simulink model "decentralized_LQR"  (R2021b)
settings: Solver=FixedStepDiscrete  StartTime=0.0  StopTime=600  FixedStep=0.5  RelTol=1e-3
values from neighbouring files (symbols this model uses):
  cte = quadrupleLoadParameters()    [decentralizedLQRComputeEqMatrices.m]
undefined symbols (not defined in the file or in its folder): cteLQR, DiscIntNeverNeededParam
libraries: sldrtlib x1
settings Model: SimulationMode=accelerator  Creator=IST  LastModifiedBy=IST

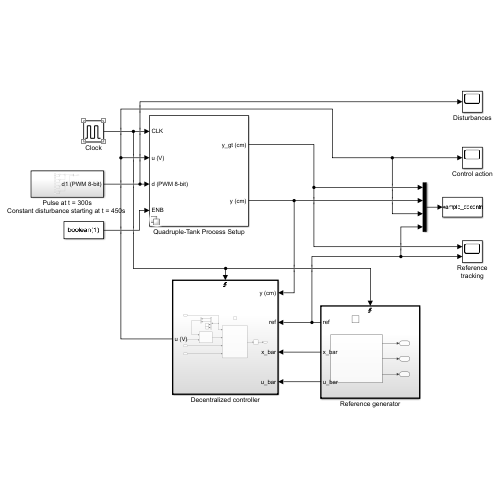
[thumbnail: Simulink's stored preview of the top-level diagram]
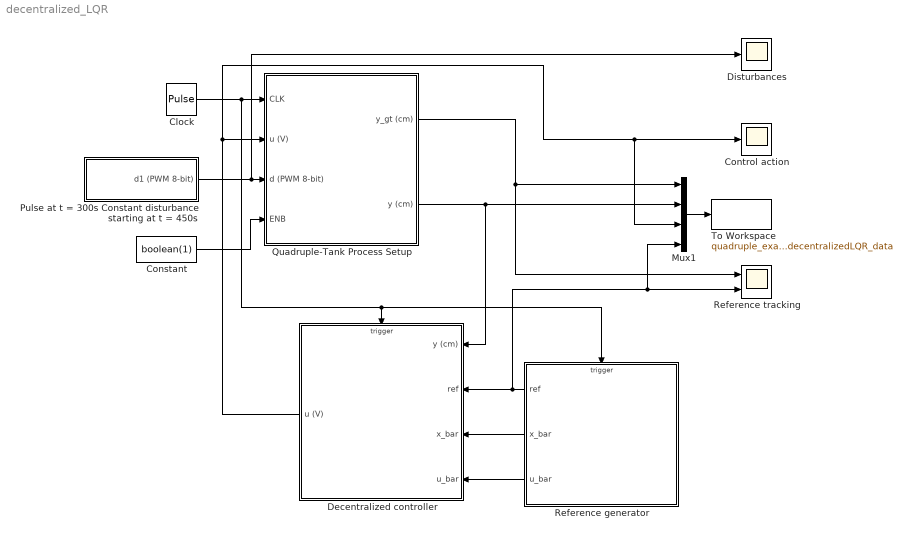
== system decentralized_LQR ==
  Clock : DiscretePulseGenerator  PulseType=Time based  Period=1  PulseWidth=50
  Constant : Constant  Priority=4  Value=boolean(1)
  Control action : Scope
      settings: Priority=20
  Decentralized controller : Subsystem  Priority=3  InitFcn=|
      | decentralizedLQRComputeEqMatrices();
      | cteLQR = decentralizedLQRLoadParameters();
  Disturbances : Scope
  Mux1 : Mux
  "Pulse at t = 300s Constant disturbance starting at t = 450s " : Subsystem
  Quadruple-Tank Process Setup : Subsystem  InitFcn=|  StopFcn=|  Variant=on
      InitFcn=|
      | % Load parameters
      | cte = quadrupleLoadParameters();
      | % Select simulation mode if unspecified
      | if ~exist('experimentalSetup')
      | experimentalSetup = false;
      | end
      | if experimentalSetup
      | if exist('arduinoPort')
      | arduino = serial(arduinoPort,...
      |                 'BaudRate',9600,...
      |                 'ByteOrder','bigEndian',...
      |                 'DataBits',8,...
      |                 'StopBits',1,...
      |                 'Terminator','');
      | arduino.Parity = 'none';
      | fopen(arduino);
      | else
      | error("Error: Arduino port undefined. Define the port in workspace variable 'arduinoPort'.");
      | end
      | end
      StopFcn=|
      | if experimentalSetup
      | fclose(arduino);
      | end
  Reference tracking : Scope  NumInputPorts=2
      settings: Priority=20
  Reference generator : Subsystem  Priority=2
  To Workspace : ToWorkspace  VariableName=quadruple_example_decentralizedLQR_data  SaveFormat=Timeseries  SampleTime=1
      settings: Priority=20
  wires:
  Quadruple-Tank Process Setup/1(y_gt (cm)) -> Reference tracking/1, Mux1/1
  Clock/1 -> Quadruple-Tank Process Setup/1(CLK), Reference generator/Trigger, Decentralized controller/Trigger
  Quadruple-Tank Process Setup/2(y (cm)) -> Decentralized controller/1(y (cm)), Mux1/2
  Mux1/1 -> To Workspace/1
  Reference generator/3(u_bar) -> Decentralized controller/4(u_bar)
  "Pulse at t = 300s Constant disturbance starting at t = 450s "/1(d1 (PWM 8-bit)) -> Disturbances/1, Quadruple-Tank Process Setup/3(d (PWM 8-bit))
  Constant/1 -> Quadruple-Tank Process Setup/4(ENB)
  Decentralized controller/1(u (V)) -> Quadruple-Tank Process Setup/2(u (V)), Mux1/3, Control action/1
  Reference generator/2(x_bar) -> Decentralized controller/3(x_bar)
  Reference generator/1(ref) -> Decentralized controller/2(ref), Mux1/4, Reference tracking/2

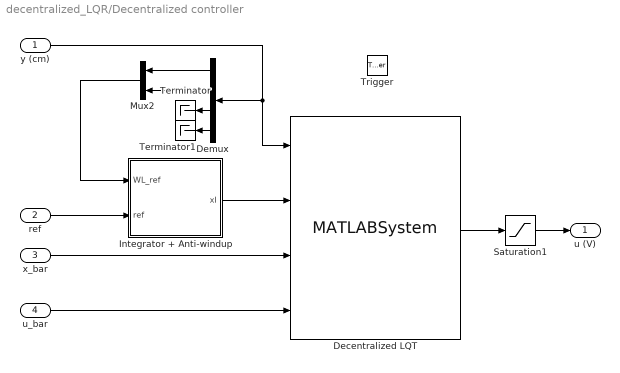
== system decentralized_LQR/Decentralized controller ==
  y (cm) : Inport
  ref : Inport  Port=2
  x_bar : Inport  Port=3
  u_bar : Inport  Port=4
  Trigger : TriggerPort  VariantControl=Variant  PortDimensions=1
  Decentralized LQT : MATLABSystem  System=controllerObj  dT=cteLQR.dT  T=cteLQR.T  d=cteLQR.d  SimulateUsing=Code generation
      mask Type: controllerObj
      mask Display:
      | disp('controllerObj');
      | port_label('input',1,'WL');
      | port_label('input',2,'xI');
      | port_label('input',3,'x_bar');
      | port_label('input',4,'u_bar');
      | port_label('output',1,'u');
  Demux : Demux
  Integrator + Anti-windup : Subsystem
  Mux2 : Mux  Inputs=2
  Saturation1 : Saturate  UpperLimit=cteLQR.uMax  LowerLimit=cteLQR.uMin
  Terminator : Terminator
  Terminator1 : Terminator
  u (V) : Outport  VectorParamsAs1DForOutWhenUnconnected=off
  wires:
  Demux/2 -> Mux2/2
  Demux/3 -> Terminator/1
  Integrator + Anti-windup/1(xI) -> Decentralized LQT/2
  Mux2/1 -> Integrator + Anti-windup/1(WL_ref)
  y (cm)/1 -> Decentralized LQT/1, Demux/1
  ref/1 -> Integrator + Anti-windup/2("ref ")
  Decentralized LQT/1 -> Saturation1/1
  Demux/1 -> Mux2/1
  Demux/4 -> Terminator1/1
  Saturation1/1 -> u (V)/1
  u_bar/1 -> Decentralized LQT/4
  x_bar/1 -> Decentralized LQT/3

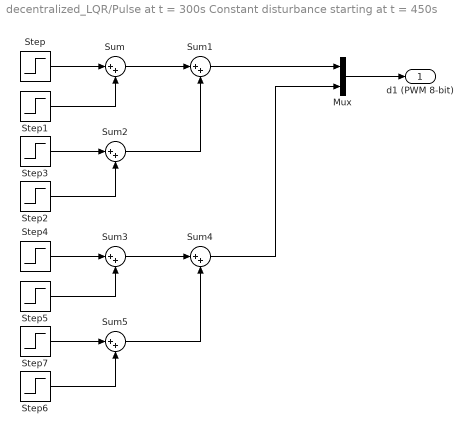
== system decentralized_LQR/Pulse at t = 300s Constant disturbance starting at t = 450s  ==
  Mux : Mux  Inputs=2
  Step : Step  Time=300  After=50  SampleTime=0
  Step1 : Step  Time=304  After=-50  SampleTime=0
  Step2 : Step  Time=451  After=-41  SampleTime=0
  Step3 : Step  Time=450  After=50  SampleTime=0
  Step4 : Step  Time=250  After=50  SampleTime=0
  Step5 : Step  Time=254  After=-50  SampleTime=0
  Step6 : Step  Time=401  After=-41  SampleTime=0
  Step7 : Step  Time=400  After=50  SampleTime=0
  Sum{,1..5} (6 alike) : Sum  Inputs=|++
  d1 (PWM 8-bit) : Outport  VectorParamsAs1DForOutWhenUnconnected=off
  wires:
  Step/1 -> Sum/1
  Step1/1 -> Sum/2
  Sum/1 -> Sum1/1
  Step3/1 -> Sum2/1
  Step2/1 -> Sum2/2
  Sum2/1 -> Sum1/2
  Sum1/1 -> Mux/1
  Step6/1 -> Sum5/2
  Step4/1 -> Sum3/1
  Sum5/1 -> Sum4/2
  Step5/1 -> Sum3/2
  Step7/1 -> Sum5/1
  Sum4/1 -> Mux/2
  Sum3/1 -> Sum4/1
  Mux/1 -> d1 (PWM 8-bit)/1

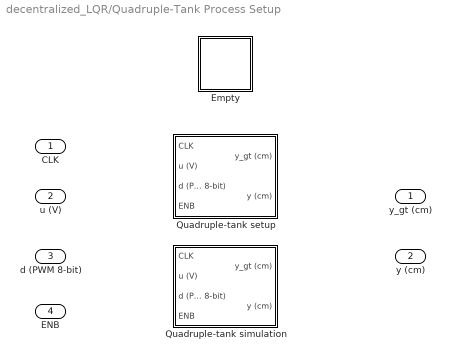
== system decentralized_LQR/Quadruple-Tank Process Setup ==
  CLK : Inport
  u (V) : Inport  Port=2
  d (PWM 8-bit) : Inport  Port=3
  ENB : Inport  Port=4
  Empty : Subsystem  VariantControl=%
  Quadruple-tank setup : Subsystem  VariantControl=experimentalSetup == true
  Quadruple-tank simulation : Subsystem  Priority=4  VariantControl=experimentalSetup == false
  y_gt (cm) : Outport  VectorParamsAs1DForOutWhenUnconnected=off
  y (cm) : Outport  Port=2  VectorParamsAs1DForOutWhenUnconnected=off

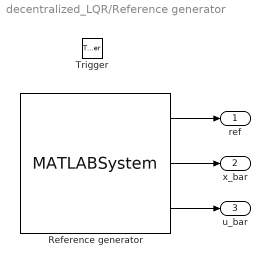
== system decentralized_LQR/Reference generator ==
  Trigger : TriggerPort  VariantControl=Variant  PortDimensions=1
  Reference generator : MATLABSystem  System=referenceGenerator  dT=cteLQR.dT  T=cteLQR.T  SimulateUsing=Code generation  Waveform1=Sin  Period1=400  Amplitude1=5  Bias1=13  Phase1=0  Waveform2=Square  Period2=300  Amplitude2=5  Bias2=13  Phase2=0
      mask Type: referenceGenerator
      mask Display:
      | disp('referenceGenerator');
      | port_label('output',1,'ref');
      | port_label('output',2,'x_bar');
      | port_label('output',3,'u_bar');
  ref : Outport  VectorParamsAs1DForOutWhenUnconnected=off
  x_bar : Outport  Port=2  VectorParamsAs1DForOutWhenUnconnected=off
  u_bar : Outport  Port=3  VectorParamsAs1DForOutWhenUnconnected=off
  wires:
  Reference generator/1 -> ref/1
  Reference generator/3 -> u_bar/1
  Reference generator/2 -> x_bar/1

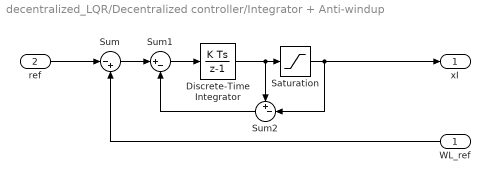
== system decentralized_LQR/Decentralized controller/Integrator + Anti-windup ==
  WL_ref : Inport
  "ref " : Inport  Port=2
  Discrete-Time Integrator : DiscreteIntegrator  SampleTime=-1  ICPrevOutput=DiscIntNeverNeededParam  ICPrevScaledInput=DiscIntNeverNeededParam
  Saturation : Saturate  UpperLimit=cteLQR.AntiWU  LowerLimit=-cteLQR.AntiWU
  Sum : Sum  Inputs=|-+
  Sum1 : Sum  Inputs=|+-
  Sum2 : Sum  Inputs=+-|
  xI : Outport  VectorParamsAs1DForOutWhenUnconnected=off
  wires:
  Discrete-Time Integrator/1 -> Sum2/1, Saturation/1
  "ref "/1 -> Sum/1
  WL_ref/1 -> Sum/2
  Sum2/1 -> Sum1/2
  Saturation/1 -> xI/1, Sum2/2
  Sum1/1 -> Discrete-Time Integrator/1
  Sum/1 -> Sum1/1

== system decentralized_LQR/Quadruple-Tank Process Setup/Empty ==

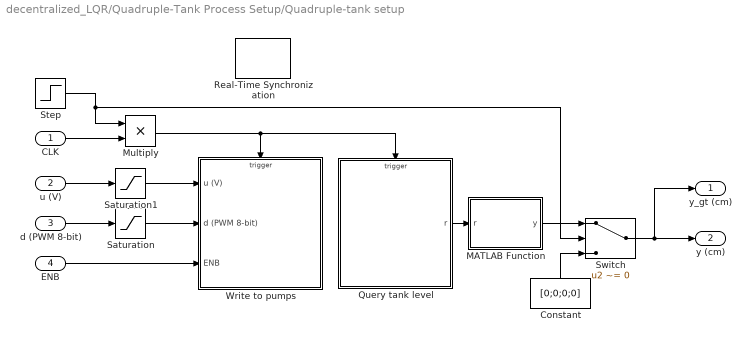
== system decentralized_LQR/Quadruple-Tank Process Setup/Quadruple-tank setup ==
  CLK : Inport
  u (V) : Inport  Port=2
  d (PWM 8-bit) : Inport  Port=3
  ENB : Inport  Port=4
  Constant : Constant  Value=[0;0;0;0]
  MATLAB Function : MATLAB Function  TreatAsAtomicUnit=on
  Multiply : Product
  Query tank level : Subsystem  Priority=1
  Real-Time Synchronization : sldrtlib/Real-Time Synchronization  Priority=5  SampleTime=0.5  MaxMissedTicks=10  ShowMissedTicks=off  YieldWhenWaiting=off
  Saturation : Saturate  UpperLimit=255  LowerLimit=0
  Saturation1 : Saturate  UpperLimit=cte.uMax  LowerLimit=cte.uMin
  Step : Step  Time=5  SampleTime=0
  Switch : Switch  Criteria=u2 ~= 0
  Write to pumps : Subsystem  Priority=100
  y_gt (cm) : Outport  VectorParamsAs1DForOutWhenUnconnected=off
  y (cm) : Outport  Port=2  VectorParamsAs1DForOutWhenUnconnected=off
  wires:
  ENB/1 -> Write to pumps/3(ENB)
  Query tank level/1(r) -> MATLAB Function/1(r)
  d (PWM 8-bit)/1 -> Saturation/1
  Saturation/1 -> Write to pumps/2(d (PWM 8-bit))
  u (V)/1 -> Saturation1/1
  Saturation1/1 -> Write to pumps/1(u (V))
  MATLAB Function/1(y) -> Switch/1
  Switch/1 -> y_gt (cm)/1, y (cm)/1
  Constant/1 -> Switch/3
  Step/1 -> Multiply/1, Switch/2
  CLK/1 -> Multiply/2
  Multiply/1 -> Write to pumps/Trigger, Query tank level/Trigger

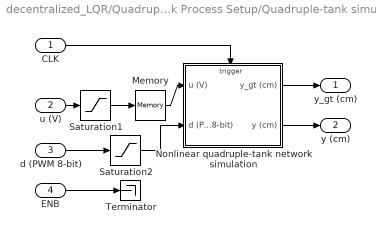
== system decentralized_LQR/Quadruple-Tank Process Setup/Quadruple-tank simulation ==
  CLK : Inport
  u (V) : Inport  Port=2
  d (PWM 8-bit) : Inport  Port=3
  ENB : Inport  Port=4
  Memory : Memory
  Nonlinear quadruple-tank network simulation : Subsystem  Priority=10
  Saturation1 : Saturate  UpperLimit=cte.uMax  LowerLimit=cte.uMin
  Saturation2 : Saturate  UpperLimit=2^8-1  LowerLimit=0
  Terminator : Terminator
  y_gt (cm) : Outport  VectorParamsAs1DForOutWhenUnconnected=off
  y (cm) : Outport  Port=2  VectorParamsAs1DForOutWhenUnconnected=off
  wires:
  CLK/1 -> Nonlinear quadruple-tank network simulation/Trigger
  Nonlinear quadruple-tank network simulation/2(y (cm)) -> y (cm)/1
  ENB/1 -> Terminator/1
  Memory/1 -> Nonlinear quadruple-tank network simulation/1(u (V))
  Nonlinear quadruple-tank network simulation/1(y_gt (cm)) -> y_gt (cm)/1
  d (PWM 8-bit)/1 -> Saturation2/1
  u (V)/1 -> Saturation1/1
  Saturation1/1 -> Memory/1
  Saturation2/1 -> Nonlinear quadruple-tank network simulation/2(d (PWM 8-bit))

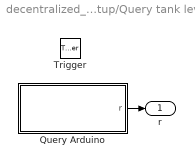
== system decentralized_LQR/Quadruple-Tank Process Setup/Quadruple-tank setup/Query tank level ==
  Trigger : TriggerPort  VariantControl=Variant  PortDimensions=1
  Query Arduino : MATLAB Function  TreatAsAtomicUnit=on
  r : Outport  VectorParamsAs1DForOutWhenUnconnected=off
  wires:
  Query Arduino/1(r) -> r/1

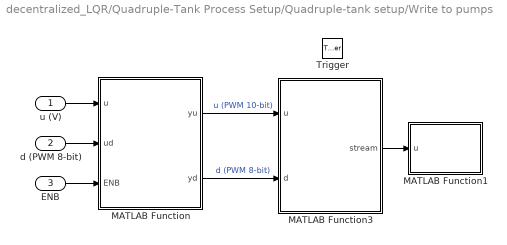
== system decentralized_LQR/Quadruple-Tank Process Setup/Quadruple-tank setup/Write to pumps ==
  u (V) : Inport
  d (PWM 8-bit) : Inport  Port=2
  ENB : Inport  Port=3
  Trigger : TriggerPort  VariantControl=Variant  PortDimensions=1
  MATLAB Function : MATLAB Function  TreatAsAtomicUnit=on
  MATLAB Function1 : MATLAB Function  TreatAsAtomicUnit=on
  MATLAB Function3 : MATLAB Function  TreatAsAtomicUnit=on
  wires:
  MATLAB Function/1(yu) -> MATLAB Function3/1(u)  "u (PWM 10-bit)"
  MATLAB Function/2(yd) -> MATLAB Function3/2(d)  "d (PWM 8-bit)"
  u (V)/1 -> MATLAB Function/1(u)
  d (PWM 8-bit)/1 -> MATLAB Function/2(ud)
  ENB/1 -> MATLAB Function/3(ENB)
  MATLAB Function3/1(stream) -> MATLAB Function1/1(u)

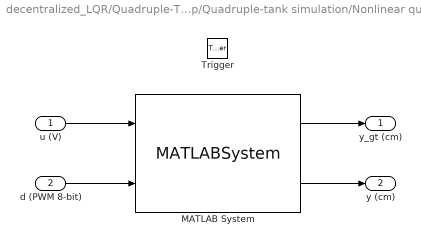
== system decentralized_LQR/Quadruple-Tank Process Setup/Quadruple-tank simulation/Nonlinear quadruple-tank network simulation ==
  u (V) : Inport
  d (PWM 8-bit) : Inport  Port=2
  Trigger : TriggerPort  VariantControl=Variant  PortDimensions=1
  MATLAB System : MATLABSystem  System=quadrupleSimObj  SimulateUsing=Interpreted execution
      mask Type: quadrupleSimObj
      mask Display:
      | disp('quadrupleSimObj');
      | port_label('input',1,'u');
      | port_label('input',2,'d');
      | port_label('output',1,'y_gt');
      | port_label('output',2,'y');
  y_gt (cm) : Outport  VectorParamsAs1DForOutWhenUnconnected=off
  y (cm) : Outport  Port=2  VectorParamsAs1DForOutWhenUnconnected=off
  wires:
  u (V)/1 -> MATLAB System/1
  MATLAB System/1 -> y_gt (cm)/1
  MATLAB System/2 -> y (cm)/1
  d (PWM 8-bit)/1 -> MATLAB System/2

== matlab function decentralized_LQR/Quadruple-Tank Process Setup/Quadruple-tank setup/Write to pumps/MATLAB Function1 ==
  data: u input
function toArduino(u)
% Find arduino serial object
coder.extrinsic('instrfind'); 
persistent arduino;
if isempty(arduino)
    arduino = instrfind('Status','open','Baud',9600);
end
% Send metadata
fprintf(arduino, "#16");
% Send actuation inputs
fwrite(arduino,u,'uint16');
end

== matlab function decentralized_LQR/Quadruple-Tank Process Setup/Quadruple-tank setup/Query tank level/Query Arduino ==
  data: r output
function r = queryArduino()
% Find arduino serial object
coder.extrinsic('instrfind'); 
persistent arduino;
if isempty(arduino)
    arduino = instrfind('Status','open','Baud',9600);
end

% Query arduino
fprintf(arduino, '$');
% Ignore metadata
fread(arduino,[4 1],'uint8');
% Read water-level data
aux = fread(arduino,[5 1],'uint16');
u = zeros(5,1);
u(5) = double(aux(5,1));
for i = 1:4
    u(i) = double(aux(i,1));
    u(i) = (u(5)-u(i))/u(i);
end
r = u(1:4);
end

== matlab function decentralized_LQR/Quadruple-Tank Process Setup/Quadruple-tank setup/Write to pumps/MATLAB Function ==
  data: u input; ud input; ENB input; yu output; cte parameter; yd output
function [yu,yd] = pwm_u(u,ud,ENB,cte)
% In u in volts
if ENB
    for i = 1:2
        u(i) = 1023*(cte.c(1,i)*cte.c(3,i)-cte.c(2,i)*cte.k(i)*u(i))/(cte.c(1,i)-cte.k(i)*u(i));
    end
    yu = u;
    yd = ud;
else
    yu = zeros(2,1);
    yd = zeros(2,1);
end

== matlab function decentralized_LQR/Quadruple-Tank Process Setup/Quadruple-tank setup/MATLAB Function ==
  data: r input; y output; cte parameter
function y = water_level(r,cte)
y = zeros(4,1);
for i = 1:4
   y(i) = r(i)*cte.dh_dr(i)+cte.h0(i);
end

== matlab function decentralized_LQR/Quadruple-Tank Process Setup/Quadruple-tank setup/Write to pumps/MATLAB Function3 ==
  data: u input; stream output; d input
function stream = packPWM10bit(u,d)
    %% Saturation 
    u(u<0) = 0;
    u(u>2^10-1) =2^10-1;
    d(d<0) = 0;
    d(d>2^8-1) =2^8-1;
    %% Pack PWM 
    stream = uint16(zeros(3,1));
    % First two actuation pump signals of 10 bits are sent individually
    stream(1:2) = uint16(round(u)); 
    % Two disturbance pump signals of 8 bits are sent together as a 16 bit
    % uint16_t
    stream(3) = uint16(round(d(1))*2^8+round(d(2)));
end
